simulink model "exp05simu"  (R2018a)
settings: Solver=VariableStepAuto  StartTime=0.0  StopTime=10.0  RelTol=1e-3
libraries: simulink x2
settings Model: Creator=SHRUTI  LastModifiedBy=SHRUTI

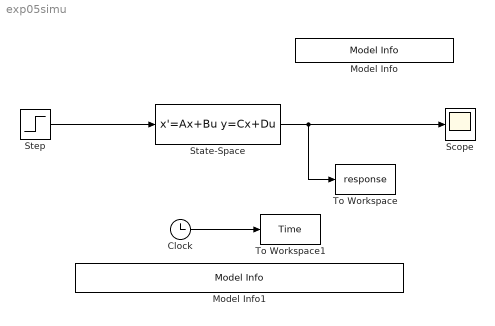
== system exp05simu ==
  Clock : Clock
  Model Info : simulink/Model-Wide Utilities/Model Info  Frame=on  DisplayStringWithTags=PRN : 17070123102  HorizontalTextAlignment=Center  LeftAlignmentValue=0.5
  Model Info1 : simulink/Model-Wide Utilities/Model Info  Frame=on  DisplayStringWithTags=SIMULINK model to visualise the State Space Representation  HorizontalTextAlignment=Center  LeftAlignmentValue=0.5
  Scope : Scope
  State-Space : StateSpace  A=[-5 1 ; -6 0]  B=[1;2]  C=[2 1]  D=0  InitialCondition=0
  Step : Step  Time=0  SampleTime=0
  To Workspace : ToWorkspace  VariableName=response  SampleTime=-1
  To Workspace1 : ToWorkspace  VariableName=Time  SampleTime=-1
  wires:
  Step/1 -> State-Space/1
  State-Space/1 -> To Workspace/1, Scope/1
  Clock/1 -> To Workspace1/1
